simulink model "TeamA_PAsqualo"  (R2020a)
settings: Solver=VariableStepAuto  StartTime=0.0  StopTime=stop_time  FixedStep=0.05  RelTol=1e-3
InitFcn:
  | main_init
values from neighbouring files (symbols this model uses):
  a1 = rho * D^4 * alpha1    (= 0.000388302366464)    [main_init.m]
  a2 = -rho * D^3 * alpha2 * (1 - omega)    (= 0.0037030698432)    [main_init.m]
  ag = [Ax Ay Az]'    [init_modello.m]
  alpha1 = 0.0113    [main_init.m]
  alpha2 = -0.0091    [main_init.m]
  areaOfInterestCorner = [42.317744;10.915136; 0]    [init_controllo.m]    (also in missionA.m = [42.317744)
  bg = [Bx By Bz]'    [init_modello.m]
  cd_pitch = 0.7    [init_modello.m]
  cd_roll = 0.04    [init_modello.m]
  cd_x = 0.4    [init_modello.m]
  cd_y = 1    [init_modello.m]
  cd_yaw = 0.7    [init_modello.m]
  cd_z = 1    [init_modello.m]
  cg = [Cx Cy Cz]'    [init_modello.m]
  D = 0.076    [main_init.m]
  dead_zone_limit = 31.5    [main_init.m]
  dg = [Dx Dy Dz]'    [init_modello.m]
  eg = [Ex Ey Ez]'    [init_modello.m]
  fg = [Fx Fy Fz]'    [init_modello.m]
  g = 9.81    [init_modello.m]
  galleggiamento = 7.6786    [init_controllo.m]
  gg = [Gx Gy Gz]'    [init_modello.m]
  H0 = 0    [init_modello.m]
  init_position = [pointP(1),pointP(2),0.15,0,0,deg2rad(alpha)]'    [init_modello.m]
  init_velocity = [0 0 0 0 0 0]'    [init_modello.m]
  initial_state_cov = blkdiag(diag(cov_gps(1,1:2)), cov_depth*eye(n_state_filter-2))    [init_navigazione.m]
  Ixx = 0.93304097392    [init_modello.m]
  Ixy = 0    [init_modello.m]
  Ixz = 0    [init_modello.m]
  Iyy = 25.58745481378    (= 25.5874548138)    [init_modello.m]
  Iyz = 0    [init_modello.m]
  Izz = 25.58745481378    (= 25.5874548138)    [init_modello.m]
  K_i_heave_div = 20    [init_controllo.m]
  K_i_heave_pos = 1    [init_controllo.m]
  K_i_heave_surf = 20    [init_controllo.m]
  K_i_heave_trans = 5    [init_controllo.m]
  K_i_heave_turn = 5    [init_controllo.m]
  K_i_pitch_div = 0    [init_controllo.m]
  K_i_pitch_pos = 0    [init_controllo.m]
  K_i_pitch_surf = 0    [init_controllo.m]
  K_i_pitch_trans = 0    [init_controllo.m]
  K_i_pitch_turn = 0    [init_controllo.m]
  K_i_roll_div = 0    [init_controllo.m]
  K_i_roll_pos = 0    [init_controllo.m]
  K_i_roll_surf = 1    [init_controllo.m]
  K_i_roll_trans = 0    [init_controllo.m]
  K_i_roll_turn = 0    [init_controllo.m]
  K_i_surge_div = 3    [init_controllo.m]
  K_i_surge_pos = 5    [init_controllo.m]
  K_i_surge_surf = 3    [init_controllo.m]
  K_i_surge_trans = 2.5    [init_controllo.m]
  K_i_surge_turn = 10    [init_controllo.m]
  K_i_sway_div = 6    [init_controllo.m]
  K_i_sway_pos = 5    [init_controllo.m]
  K_i_sway_surf = 3    [init_controllo.m]
  K_i_sway_trans = 6    [init_controllo.m]
  K_i_sway_turn = 50    [init_controllo.m]
  K_i_yaw_div = 0    [init_controllo.m]
  K_i_yaw_pos = 1    [init_controllo.m]
  K_i_yaw_surf = 0    [init_controllo.m]
  K_i_yaw_trans = 20    [init_controllo.m]
  K_p_heave_div = 200    [init_controllo.m]
  K_p_heave_pos = 350    [init_controllo.m]
  K_p_heave_surf = 200    [init_controllo.m]
  K_p_heave_trans = 200    [init_controllo.m]
  K_p_heave_turn = 200    [init_controllo.m]
  K_p_phi_div = 0.15    [init_controllo.m]
  K_p_phi_pos = 0.1    [init_controllo.m]
  K_p_phi_surf = 0.15    [init_controllo.m]
  K_p_phi_trans = 0.1    [init_controllo.m]
  K_p_phi_turn = 0.1    [init_controllo.m]
  K_p_pitch_div = 50    [init_controllo.m]
  K_p_pitch_pos = 25    [init_controllo.m]
  K_p_pitch_surf = 50    [init_controllo.m]
  K_p_pitch_trans = 25    [init_controllo.m]
  K_p_pitch_turn = 25    [init_controllo.m]
  K_p_psi_div = 0.3    [init_controllo.m]
  K_p_psi_pos = 0.25    [init_controllo.m]
  K_p_psi_surf = 0.3    [init_controllo.m]
  K_p_psi_trans = 0.2    [init_controllo.m]
  K_p_roll_div = 10    [init_controllo.m]
  K_p_roll_pos = 4    [init_controllo.m]
  K_p_roll_surf = 10    [init_controllo.m]
  K_p_roll_trans = 4    [init_controllo.m]
  K_p_roll_turn = 4    [init_controllo.m]
  K_p_surge_div = 80    [init_controllo.m]
  K_p_surge_pos = 34.5    [init_controllo.m]
  K_p_surge_surf = 80    [init_controllo.m]
  K_p_surge_trans = 40    [init_controllo.m]
  K_p_surge_turn = 150    [init_controllo.m]
  K_p_sway_div = 100    [init_controllo.m]
  K_p_sway_pos = 90    [init_controllo.m]
  K_p_sway_surf = 80    [init_controllo.m]
  K_p_sway_trans = 90    [init_controllo.m]
  K_p_sway_turn = 200    [init_controllo.m]
  K_p_th_div = 0.3    [init_controllo.m]
  K_p_th_pos = 0.1    [init_controllo.m]
  K_p_th_surf = 0.3    [init_controllo.m]
  K_p_th_trans = 0.1    [init_controllo.m]
  K_p_th_turn = 0.1    [init_controllo.m]
  K_p_x_div = 0.12    [init_controllo.m]
  K_p_x_pos = 0.12    [init_controllo.m]
  K_p_x_surf = 0.12    [init_controllo.m]
  K_p_y_div = 0.6    [init_controllo.m]
  K_p_y_pos = 0.34    [init_controllo.m]
  K_p_y_surf = 0.1    [init_controllo.m]
  K_p_y_trans = 0.3    [init_controllo.m]
  K_p_y_turn = 0.3    [init_controllo.m]
  K_p_yaw_div = 70    [init_controllo.m]
  K_p_yaw_pos = 20    [init_controllo.m]
  K_p_yaw_surf = 70    [init_controllo.m]
  K_p_yaw_trans = 160    [init_controllo.m]
  K_p_z_div = 0.35    [init_controllo.m]
  K_p_z_pos = 0.2    [init_controllo.m]
  K_p_z_surf = 0.35    [init_controllo.m]
  K_p_z_trans = 0.7    [init_controllo.m]
  K_p_z_turn = 0.7    [init_controllo.m]
  Kadd = 0    [init_modello.m]
  m = 106    [init_modello.m]
  Madd = -((((1/5)*(b^2-a^2)^2))*(alpha_0-beta_0))/((((2*(b^2-a^2)^2))+(b^2-a^2)^2)*(alpha_0-beta_0)*m)    [init_modello.m]
  ... (+59 more)
undefined symbols (not defined in the file or in its folder): DiscIntNeverNeededParam, initial_state
libraries: simulink x2, vrlib x1
(part 3 of 5)

== system TeamA_PAsqualo/controller/surfacing controller/sway_controller/Sway PID controller ==
  enable : Inport
  references : Inport  Port=2
  "estimated measures " : Inport  Port=3
  Constant : Constant
  Constant1 : Constant  Value=0
  Discrete-Time Integrator : DiscreteIntegrator  ExternalReset=falling  SampleTime=0.1  ICPrevOutput=DiscIntNeverNeededParam  ICPrevScaledInput=DiscIntNeverNeededParam
  K_i_sway_surf : Gain  Gain=K_i_sway_surf
  K_p_sway_surf : Gain  Gain=K_p_sway_surf
  K_p_y_surf : Gain  Gain=K_p_y_surf
  Sum2 : Sum
  Switch : Switch  Threshold=1
  compute_position_errors : MATLAB Function  TreatAsAtomicUnit=on
  compute_velocity_error : MATLAB Function  TreatAsAtomicUnit=on
  Y : Outport
  wires:
  references/1 -> compute_position_errors/2(ref)
  compute_position_errors/1(err_pos) -> K_p_y_surf/1  "err_y"
  K_p_y_surf/1 -> compute_velocity_error/2(v_des)
  "estimated measures "/1 -> compute_velocity_error/3(est_meas), compute_position_errors/3(est_state)
  K_i_sway_surf/1 -> Discrete-Time Integrator/1
  K_p_sway_surf/1 -> Sum2/1
  Sum2/1 -> Y/1
  compute_velocity_error/1(err_vel) -> K_i_sway_surf/1, K_p_sway_surf/1  "err_vel"
  Discrete-Time Integrator/1 -> Sum2/2
  Switch/1 -> Discrete-Time Integrator/2
  enable/1 -> Switch/2, compute_velocity_error/1(enable), compute_position_errors/1(enable)
  Constant1/1 -> Switch/3
  Constant/1 -> Switch/1

== system TeamA_PAsqualo/controller/surfacing controller/yaw_controller/Yaw PID controller ==
  enable : Inport
  references : Inport  Port=2
  "estimated measures " : Inport  Port=3
  Constant : Constant
  Constant1 : Constant  Value=0
  Discrete-Time Integrator : DiscreteIntegrator  ExternalReset=falling  SampleTime=0.1  ICPrevOutput=DiscIntNeverNeededParam  ICPrevScaledInput=DiscIntNeverNeededParam
  K_i_yaw_surf : Gain  Gain=K_i_yaw_surf
  K_p_psi_surf : Gain  Gain=K_p_psi_surf
  K_p_yaw_surf : Gain  Gain=K_p_yaw_surf
  Sum2 : Sum
  Switch : Switch  Threshold=1
  compute_orientation_errors : MATLAB Function  TreatAsAtomicUnit=on
  compute_velocity_error : MATLAB Function  TreatAsAtomicUnit=on
  N : Outport
  wires:
  references/1 -> compute_orientation_errors/2(ref)
  "estimated measures "/1 -> compute_velocity_error/3(est_meas), compute_orientation_errors/3(est_state)
  compute_orientation_errors/1(err_orient) -> K_p_psi_surf/1  "err_orient"
  K_p_psi_surf/1 -> compute_velocity_error/2(v_des)
  Sum2/1 -> N/1
  Discrete-Time Integrator/1 -> Sum2/2
  K_i_yaw_surf/1 -> Discrete-Time Integrator/1
  K_p_yaw_surf/1 -> Sum2/1
  compute_velocity_error/1(err_vel) -> K_i_yaw_surf/1, K_p_yaw_surf/1  "err_vel"
  Switch/1 -> Discrete-Time Integrator/2
  enable/1 -> Switch/2, compute_velocity_error/1(enable), compute_orientation_errors/1(enable)
  Constant1/1 -> Switch/3
  Constant/1 -> Switch/1

== system TeamA_PAsqualo/controller/transect controller/heave_controller/Heave PID controller ==
  enable : Inport
  references : Inport  Port=2
  "estimated measures " : Inport  Port=3
  Constant : Constant  Value=galleggiamento
  Constant1 : Constant
  Constant2 : Constant  Value=0
  Discrete-Time Integrator : DiscreteIntegrator  ExternalReset=falling  InitialConditionSource=external  SampleTime=0.1  ICPrevOutput=DiscIntNeverNeededParam  ICPrevScaledInput=DiscIntNeverNeededParam
  K_i_heave_trans : Gain  Gain=K_i_heave_trans
  K_p_heave_trans : Gain  Gain=K_p_heave_trans
  K_p_z_trans : Gain  Gain=K_p_z_trans
  Sum2 : Sum
  Switch : Switch  Threshold=1
  compute_position_errors : MATLAB Function  TreatAsAtomicUnit=on
  compute_velocity_error : MATLAB Function  TreatAsAtomicUnit=on
  Z : Outport
  wires:
  "estimated measures "/1 -> compute_velocity_error/3(est_meas), compute_position_errors/3(est_state)
  K_p_z_trans/1 -> compute_velocity_error/2(v_des)
  compute_position_errors/1(err_pos) -> K_p_z_trans/1  "err_vect"
  references/1 -> compute_position_errors/2(ref)
  Sum2/1 -> Z/1
  Discrete-Time Integrator/1 -> Sum2/2
  K_p_heave_trans/1 -> Sum2/1
  K_i_heave_trans/1 -> Discrete-Time Integrator/1
  compute_velocity_error/1(err_vel) -> K_i_heave_trans/1, K_p_heave_trans/1  "err_vel"
  Constant/1 -> Discrete-Time Integrator/3
  Switch/1 -> Discrete-Time Integrator/2
  enable/1 -> Switch/2, compute_velocity_error/1(enable), compute_position_errors/1(enable)
  Constant2/1 -> Switch/3
  Constant1/1 -> Switch/1

== system TeamA_PAsqualo/controller/transect controller/pitch_controller/Pitch PID controller ==
  enable : Inport
  references : Inport  Port=2
  "estimated measures " : Inport  Port=3
  Constant : Constant
  Constant1 : Constant  Value=0
  Discrete-Time Integrator : DiscreteIntegrator  ExternalReset=falling  SampleTime=0.1  ICPrevOutput=DiscIntNeverNeededParam  ICPrevScaledInput=DiscIntNeverNeededParam
  K_i_pitch_trans : Gain  Gain=K_i_pitch_trans
  K_p_pitch_trans : Gain  Gain=K_p_pitch_trans
  K_p_th_trans : Gain  Gain=K_p_th_trans
  Sum2 : Sum
  Switch : Switch  Threshold=1
  compute_orientation_errors : MATLAB Function  TreatAsAtomicUnit=on
  compute_velocity_error : MATLAB Function  TreatAsAtomicUnit=on
  M : Outport
  wires:
  references/1 -> compute_orientation_errors/2(ref)
  K_p_th_trans/1 -> compute_velocity_error/2(v_des)
  "estimated measures "/1 -> compute_velocity_error/3(est_meas), compute_orientation_errors/3(est_state)
  compute_orientation_errors/1(err_orient) -> K_p_th_trans/1  "err_orient"
  Sum2/1 -> M/1
  Discrete-Time Integrator/1 -> Sum2/2
  K_p_pitch_trans/1 -> Sum2/1
  K_i_pitch_trans/1 -> Discrete-Time Integrator/1
  compute_velocity_error/1(err_vel) -> K_i_pitch_trans/1, K_p_pitch_trans/1  "err_vel"
  Switch/1 -> Discrete-Time Integrator/2
  enable/1 -> Switch/2, compute_velocity_error/1(enable), compute_orientation_errors/1(enable)
  Constant1/1 -> Switch/3
  Constant/1 -> Switch/1

== system TeamA_PAsqualo/controller/transect controller/roll_controller/Roll PID controller ==
  enable : Inport
  references : Inport  Port=2
  "estimated measures " : Inport  Port=3
  Constant : Constant
  Constant1 : Constant  Value=0
  Discrete-Time Integrator : DiscreteIntegrator  ExternalReset=falling  SampleTime=0.1  ICPrevOutput=DiscIntNeverNeededParam  ICPrevScaledInput=DiscIntNeverNeededParam
  K_i_roll_trans : Gain  Gain=K_i_roll_trans
  K_p_phi_trans : Gain  Gain=K_p_phi_trans
  K_p_roll_trans : Gain  Gain=K_p_roll_trans
  Sum2 : Sum
  Switch : Switch  Threshold=1
  compute_orientation_errors : MATLAB Function  TreatAsAtomicUnit=on
  compute_velocity_error : MATLAB Function  TreatAsAtomicUnit=on
  tau_roll : Outport
  wires:
  "estimated measures "/1 -> compute_velocity_error/3(est_meas), compute_orientation_errors/3(est_state)
  K_p_phi_trans/1 -> compute_velocity_error/2(v_des)
  compute_orientation_errors/1(err_orient) -> K_p_phi_trans/1  "err_orient"
  references/1 -> compute_orientation_errors/2(ref)
  Sum2/1 -> tau_roll/1
  Discrete-Time Integrator/1 -> Sum2/2
  K_p_roll_trans/1 -> Sum2/1
  K_i_roll_trans/1 -> Discrete-Time Integrator/1
  compute_velocity_error/1(err_vel) -> K_p_roll_trans/1, K_i_roll_trans/1  "err_vel"
  Switch/1 -> Discrete-Time Integrator/2
  Constant1/1 -> Switch/3
  Constant/1 -> Switch/1
  enable/1 -> Switch/2, compute_velocity_error/1(enable), compute_orientation_errors/1(enable)

== system TeamA_PAsqualo/controller/transect controller/surge_controller/Surge PID controller ==
  enable : Inport
  ref : Inport  Port=2
  est_meas : Inport  Port=3
  " compute_velocity_error" : MATLAB Function  TreatAsAtomicUnit=on
  Constant : Constant
  Constant1 : Constant  Value=0
  Discrete-Time Integrator : DiscreteIntegrator  ExternalReset=falling  SampleTime=0.1  ICPrevOutput=DiscIntNeverNeededParam  ICPrevScaledInput=DiscIntNeverNeededParam
  K_i_surge_trans : Gain  Gain=K_i_surge_trans
  K_p_surge_trans : Gain  Gain=K_p_surge_trans
  Scope : Scope
  Sum2 : Sum
  Switch : Switch  Threshold=1
  X : Outport
  wires:
  est_meas/1 -> " compute_velocity_error"/3(est_meas)
  ref/1 -> " compute_velocity_error"/2(ref)
  " compute_velocity_error"/1(err_vel) -> K_i_surge_trans/1, K_p_surge_trans/1  "err_vel"
  K_p_surge_trans/1 -> Sum2/1
  Sum2/1 -> Scope/1, X/1  "X"
  K_i_surge_trans/1 -> Discrete-Time Integrator/1
  Discrete-Time Integrator/1 -> Sum2/2
  Switch/1 -> Discrete-Time Integrator/2
  enable/1 -> Switch/2, " compute_velocity_error"/1(enable)
  Constant1/1 -> Switch/3
  Constant/1 -> Switch/1

== system TeamA_PAsqualo/controller/transect controller/sway_controller/Sway PID controller ==
  enable : Inport
  references : Inport  Port=2
  "estimated measures " : Inport  Port=3
  Constant : Constant
  Constant1 : Constant  Value=0
  Discrete-Time Integrator : DiscreteIntegrator  ExternalReset=falling  SampleTime=0.1  LimitOutput=on  ICPrevOutput=DiscIntNeverNeededParam  ICPrevScaledInput=DiscIntNeverNeededParam
  K_i_sway_trans : Gain  Gain=K_i_sway_trans
  K_p_sway_trans : Gain  Gain=K_p_sway_trans
  K_p_y_trans : Gain  Gain=K_p_y_trans
  Scope : Scope
  Sum2 : Sum
  Switch : Switch  Threshold=1
  compute_position_errors : MATLAB Function  TreatAsAtomicUnit=on
  compute_velocity_error : MATLAB Function  TreatAsAtomicUnit=on
  Y : Outport
  wires:
  references/1 -> compute_position_errors/2(ref)
  compute_position_errors/1(err_pos) -> K_p_y_trans/1  "err_vect"
  K_p_y_trans/1 -> compute_velocity_error/2(v_des)
  "estimated measures "/1 -> compute_velocity_error/3(est_meas), compute_position_errors/3(est_state)
  compute_velocity_error/1(err_vel) -> K_i_sway_trans/1, K_p_sway_trans/1  "err_vel"
  Discrete-Time Integrator/1 -> Scope/1, Sum2/2
  K_i_sway_trans/1 -> Discrete-Time Integrator/1
  Sum2/1 -> Y/1
  K_p_sway_trans/1 -> Sum2/1
  Switch/1 -> Discrete-Time Integrator/2
  enable/1 -> Switch/2, compute_velocity_error/1(enable), compute_position_errors/1(enable)
  Constant1/1 -> Switch/3
  Constant/1 -> Switch/1

== system TeamA_PAsqualo/controller/transect controller/yaw_controller/Yaw PID controller ==
  enable : Inport
  references : Inport  Port=2
  "estimated measures " : Inport  Port=3
  Constant : Constant
  Constant1 : Constant  Value=0
  Discrete-Time Integrator : DiscreteIntegrator  ExternalReset=falling  SampleTime=0.1  ICPrevOutput=DiscIntNeverNeededParam  ICPrevScaledInput=DiscIntNeverNeededParam
  K_i_yaw_trans : Gain  Gain=K_i_yaw_trans
  K_p_psi_trans : Gain  Gain=K_p_psi_trans
  K_p_yaw_trans : Gain  Gain=K_p_yaw_trans
  Sum2 : Sum
  Switch : Switch  Threshold=1
  compute_orientation_errors : MATLAB Function  TreatAsAtomicUnit=on
  compute_velocity_error : MATLAB Function  TreatAsAtomicUnit=on
  N : Outport
  wires:
  references/1 -> compute_orientation_errors/2(ref)
  "estimated measures "/1 -> compute_velocity_error/3(est_meas), compute_orientation_errors/3(est_state)
  compute_orientation_errors/1(err_orient) -> K_p_psi_trans/1  "err_orient"
  K_p_psi_trans/1 -> compute_velocity_error/2(v_des)
  Sum2/1 -> N/1
  Discrete-Time Integrator/1 -> Sum2/2
  K_p_yaw_trans/1 -> Sum2/1
  K_i_yaw_trans/1 -> Discrete-Time Integrator/1
  compute_velocity_error/1(err_vel) -> K_i_yaw_trans/1, K_p_yaw_trans/1  "err_vel"
  Switch/1 -> Discrete-Time Integrator/2
  enable/1 -> Switch/2, compute_velocity_error/1(enable), compute_orientation_errors/1(enable)
  Constant1/1 -> Switch/3
  Constant/1 -> Switch/1

== system TeamA_PAsqualo/controller/turning controller/heave_controller/Heave PID controller ==
  enable : Inport
  references : Inport  Port=2
  "estimated measures " : Inport  Port=3
  Constant : Constant  Value=galleggiamento
  Constant1 : Constant
  Constant2 : Constant  Value=0
  Discrete-Time Integrator : DiscreteIntegrator  ExternalReset=falling  InitialConditionSource=external  SampleTime=0.1  ICPrevOutput=DiscIntNeverNeededParam  ICPrevScaledInput=DiscIntNeverNeededParam
  K_i_heave_turn : Gain  Gain=K_i_heave_turn
  K_p_heave_turn : Gain  Gain=K_p_heave_turn
  K_p_z_turn : Gain  Gain=K_p_z_turn
  Sum2 : Sum
  Switch : Switch  Threshold=1
  compute_position_errors : MATLAB Function  TreatAsAtomicUnit=on
  compute_velocity_error : MATLAB Function  TreatAsAtomicUnit=on
  Z : Outport
  wires:
  "estimated measures "/1 -> compute_velocity_error/3(est_meas), compute_position_errors/3(est_state)
  K_p_z_turn/1 -> compute_velocity_error/2(v_des)
  compute_position_errors/1(err_pos) -> K_p_z_turn/1  "err_vect"
  references/1 -> compute_position_errors/2(ref)
  K_p_heave_turn/1 -> Sum2/1
  K_i_heave_turn/1 -> Discrete-Time Integrator/1
  Discrete-Time Integrator/1 -> Sum2/2
  Sum2/1 -> Z/1
  compute_velocity_error/1(err_vel) -> K_i_heave_turn/1, K_p_heave_turn/1  "err_vel"
  Constant/1 -> Discrete-Time Integrator/3
  Switch/1 -> Discrete-Time Integrator/2
  enable/1 -> Switch/2, compute_velocity_error/1(enable), compute_position_errors/1(enable)
  Constant2/1 -> Switch/3
  Constant1/1 -> Switch/1

== system TeamA_PAsqualo/controller/turning controller/pitch_controller/Pitch PID controller ==
  enable : Inport
  references : Inport  Port=2
  "estimated measures " : Inport  Port=3
  Constant : Constant
  Constant1 : Constant  Value=0
  Discrete-Time Integrator : DiscreteIntegrator  ExternalReset=falling  SampleTime=0.1  ICPrevOutput=DiscIntNeverNeededParam  ICPrevScaledInput=DiscIntNeverNeededParam
  K_i_pitch_turn : Gain  Gain=K_i_pitch_turn
  K_p_pitch_turn : Gain  Gain=K_p_pitch_turn
  K_p_th_turn : Gain  Gain=K_p_th_turn
  Sum2 : Sum
  Switch : Switch  Threshold=1
  compute_orientation_errors : MATLAB Function  TreatAsAtomicUnit=on
  compute_velocity_error : MATLAB Function  TreatAsAtomicUnit=on
  M : Outport
  wires:
  references/1 -> compute_orientation_errors/2(ref)
  K_p_th_turn/1 -> compute_velocity_error/2(v_des)
  "estimated measures "/1 -> compute_velocity_error/3(est_meas), compute_orientation_errors/3(est_state)
  compute_orientation_errors/1(err_orient) -> K_p_th_turn/1  "err_orient"
  Sum2/1 -> M/1
  compute_velocity_error/1(err_vel) -> K_i_pitch_turn/1, K_p_pitch_turn/1  "err_vel"
  Discrete-Time Integrator/1 -> Sum2/2
  K_p_pitch_turn/1 -> Sum2/1
  K_i_pitch_turn/1 -> Discrete-Time Integrator/1
  Switch/1 -> Discrete-Time Integrator/2
  enable/1 -> Switch/2, compute_velocity_error/1(enable), compute_orientation_errors/1(enable)
  Constant1/1 -> Switch/3
  Constant/1 -> Switch/1

== system TeamA_PAsqualo/controller/turning controller/roll_controller/Roll PID controller ==
  enable : Inport
  references : Inport  Port=2
  "estimated measures " : Inport  Port=3
  Constant : Constant
  Constant1 : Constant  Value=0
  Discrete-Time Integrator : DiscreteIntegrator  ExternalReset=falling  SampleTime=0.1  ICPrevOutput=DiscIntNeverNeededParam  ICPrevScaledInput=DiscIntNeverNeededParam
  K_i_roll_turn : Gain  Gain=K_i_roll_turn
  K_p_phi_turn : Gain  Gain=K_p_phi_turn
  K_p_roll_turn : Gain  Gain=K_p_roll_turn
  Sum2 : Sum
  Switch : Switch  Threshold=1
  compute_orientation_errors : MATLAB Function  TreatAsAtomicUnit=on
  compute_velocity_error : MATLAB Function  TreatAsAtomicUnit=on
  K : Outport
  wires:
  "estimated measures "/1 -> compute_velocity_error/3(est_meas), compute_orientation_errors/3(est_state)
  K_p_phi_turn/1 -> compute_velocity_error/2(v_des)
  compute_orientation_errors/1(err_orient) -> K_p_phi_turn/1  "err_orient"
  references/1 -> compute_orientation_errors/2(ref)
  Sum2/1 -> K/1
  compute_velocity_error/1(err_vel) -> K_i_roll_turn/1, K_p_roll_turn/1  "err_vel"
  Discrete-Time Integrator/1 -> Sum2/2
  K_p_roll_turn/1 -> Sum2/1
  K_i_roll_turn/1 -> Discrete-Time Integrator/1
  Switch/1 -> Discrete-Time Integrator/2
  enable/1 -> Switch/2, compute_velocity_error/1(enable), compute_orientation_errors/1(enable)
  Constant1/1 -> Switch/3
  Constant/1 -> Switch/1

== system TeamA_PAsqualo/controller/turning controller/surge_controller/Surge PID controller ==
  enable : Inport
  ref : Inport  Port=2
  est_meas : Inport  Port=3
  " compute_velocity_error" : MATLAB Function  TreatAsAtomicUnit=on
  Constant : Constant
  Constant1 : Constant  Value=0
  Constant2 : Constant  Value=turning_surge
  Discrete-Time Integrator : DiscreteIntegrator  ExternalReset=falling  InitialConditionSource=external  SampleTime=0.1  ICPrevOutput=DiscIntNeverNeededParam  ICPrevScaledInput=DiscIntNeverNeededParam
  K_i_surge_turn : Gain  Gain=K_i_surge_turn
  K_p_surge_turn : Gain  Gain=K_p_surge_turn
  Scope : Scope
  Sum2 : Sum
  Switch : Switch  Threshold=1
  X : Outport
  wires:
  est_meas/1 -> " compute_velocity_error"/3(est_meas)
  ref/1 -> " compute_velocity_error"/2(ref)
  Sum2/1 -> Scope/1, X/1
  Discrete-Time Integrator/1 -> Sum2/2
  K_p_surge_turn/1 -> Sum2/1
  K_i_surge_turn/1 -> Discrete-Time Integrator/1
  " compute_velocity_error"/1(err_vel) -> K_i_surge_turn/1, K_p_surge_turn/1  "err_vel"
  Switch/1 -> Discrete-Time Integrator/2
  enable/1 -> Switch/2, " compute_velocity_error"/1(enable)
  Constant1/1 -> Switch/3
  Constant/1 -> Switch/1
  Constant2/1 -> Discrete-Time Integrator/3

== system TeamA_PAsqualo/controller/turning controller/sway_controller/Sway PID controller ==
  enable : Inport
  references : Inport  Port=2
  "estimated measures " : Inport  Port=3
  Constant : Constant
  Constant1 : Constant  Value=0
  Discrete-Time Integrator : DiscreteIntegrator  ExternalReset=falling  SampleTime=0.1  ICPrevOutput=DiscIntNeverNeededParam  ICPrevScaledInput=DiscIntNeverNeededParam
  K_i_sway_turn : Gain  Gain=K_i_sway_turn
  K_p_sway_turn : Gain  Gain=K_p_sway_turn
  K_p_y_turn : Gain  Gain=K_p_y_turn
  Scope : Scope
  Sum2 : Sum
  Switch : Switch  Threshold=1
  compute_position_errors : MATLAB Function  TreatAsAtomicUnit=on
  compute_velocity_error : MATLAB Function  TreatAsAtomicUnit=on
  Y : Outport
  wires:
  references/1 -> compute_position_errors/2(ref)
  compute_position_errors/1(err_pos) -> K_p_y_turn/1  "err_vect"
  K_p_y_turn/1 -> compute_velocity_error/2(v_des)
  "estimated measures "/1 -> compute_velocity_error/3(est_meas), compute_position_errors/3(est_state)
  K_p_sway_turn/1 -> Sum2/1
  K_i_sway_turn/1 -> Discrete-Time Integrator/1
  Discrete-Time Integrator/1 -> Scope/1, Sum2/2
  compute_velocity_error/1(err_vel) -> K_i_sway_turn/1, K_p_sway_turn/1  "err_vel"
  Sum2/1 -> Y/1
  Switch/1 -> Discrete-Time Integrator/2
  enable/1 -> Switch/2, compute_velocity_error/1(enable), compute_position_errors/1(enable)
  Constant1/1 -> Switch/3
  Constant/1 -> Switch/1

== system TeamA_PAsqualo/controller/turning controller/yaw_controller/Yaw PID controller ==
  enable : Inport
  ref : Inport  Port=2
  est_meas : Inport  Port=3
  Constant2 : Constant
  Constant3 : Constant  Value=0
  Discrete-Time Integrator1 : DiscreteIntegrator  ExternalReset=falling  SampleTime=0.1  ICPrevOutput=DiscIntNeverNeededParam  ICPrevScaledInput=DiscIntNeverNeededParam
  K_i_yaw_trans : Gain  Gain=K_i_yaw_trans
  K_p_psi_trans : Gain  Gain=K_p_psi_trans
  K_p_yaw_trans : Gain  Gain=K_p_yaw_trans
  Sum1 : Sum
  Switch1 : Switch  Threshold=1
  compute_orientation_errors : MATLAB Function  TreatAsAtomicUnit=on
  compute_velocity_error : MATLAB Function  TreatAsAtomicUnit=on
  N : Outport
  wires:
  Constant3/1 -> Switch1/3
  Constant2/1 -> Switch1/1
  K_p_psi_trans/1 -> compute_velocity_error/2(v_des)
  Switch1/1 -> Discrete-Time Integrator1/2
  compute_velocity_error/1(err_vel) -> K_i_yaw_trans/1, K_p_yaw_trans/1  "err_vel"
  enable/1 -> Switch1/2, compute_velocity_error/1(enable), compute_orientation_errors/1(enable)
  K_i_yaw_trans/1 -> Discrete-Time Integrator1/1
  compute_orientation_errors/1(err_orient) -> K_p_psi_trans/1  "err_orient"
  est_meas/1 -> compute_orientation_errors/3(est_state), compute_velocity_error/3(est_meas)
  K_p_yaw_trans/1 -> Sum1/1
  ref/1 -> compute_orientation_errors/2(ref)
  Discrete-Time Integrator1/1 -> Sum1/2
  Sum1/1 -> N/1

== matlab function TeamA_PAsqualo/Vehicle Model/J1 computation ==
  data: eta input; J1 output
function J1 = fcn(eta)
phi = eta(4);
theta = eta(5);
psi = eta(6);
Rx = [1 0 0;0 cos(phi) sin(phi);0 -sin(phi) cos(phi)];
Ry = [cos(theta) 0 -sin(theta);0 1 0;sin(theta) 0 cos(theta)];
Rz = [cos(psi) sin(psi) 0;-sin(psi) cos(psi) 0; 0 0 1];
J1 = Rz'*Ry'*Rx';
end

== matlab function TeamA_PAsqualo/Vehicle Model/ni_dot computation ==
  data: M_times_nir_dot input double size=[6 1]; nir_dot output double size=[6 1]; M_inv parameter
function nir_dot = fcn(M_times_nir_dot, M_inv)
nir_dot = M_inv * M_times_nir_dot;
end

== matlab function TeamA_PAsqualo/Vehicle Model/ni_to_eta_dot ==
  data: J input; ni_abs input; eta_dot output
function eta_dot = fcn(J,ni_abs)
eta_dot = J*ni_abs;
end

== matlab function TeamA_PAsqualo/Sensors and Environment Models /Global Positioning System/WGS84toNed  ==
  data: posizione input; posizione_NED output
function posizione_NED = wgs84toNed(posizione)

coder.extrinsic('evalin', 'wgs84Ellipsoid', 'geodetic2ned');
NED_origin = [0;0;0];
posizione_NED  = [0;0;0];
NED_origin = evalin('base', 'NED_origin');
[a, b, c] = geodetic2ned(posizione(1), posizione(2), posizione(3), NED_origin(1), NED_origin(2), NED_origin(3), wgs84Ellipsoid);
posizione_NED = [a; b; posizione(3)];

end

== matlab function TeamA_PAsqualo/Sensors and Environment Models /Profondimetro/WGS84toNed  ==
  data: posizione input; posizione_NED output
function posizione_NED = wgs84toNed(posizione)

coder.extrinsic('evalin', 'wgs84Ellipsoid', 'geodetic2ned');
NED_origin = [0;0;0];
posizione_NED  = [0;0;0];
NED_origin = evalin('base', 'NED_origin');
[a, b, c] = geodetic2ned(posizione(1), posizione(2), posizione(3), NED_origin(1), NED_origin(2), NED_origin(3), wgs84Ellipsoid);
posizione_NED = [a; b; posizione(3)];

end

== matlab function TeamA_PAsqualo/Sensors and Environment Models /Sonar_down/MATLAB Function ==
  data: posizione input; p_sonar_ned output; orientazione input; s_versor_ned output; tilt input; p_sonar_body input
function [p_sonar_ned, s_versor_ned] = rot_body_ned(posizione,orientazione,tilt,p_sonar_body)
   
 roll = orientazione(1);
 pitch = orientazione(2);
 yaw = orientazione(3);
 xNorth = posizione(1);
 yEast = posizione(2);
 zDown = posizione(3);
 Rx = [1 0 0; 0 cos(roll) -sin(roll); 0 sin(roll) cos(roll)];
 Ry = [cos(pitch) 0 sin(pitch); 0 1 0; -sin(pitch) 0 cos(pitch)];
 Rz = [cos(yaw) -sin(yaw) 0; sin(yaw) cos(yaw) 0; 0 0 1];
 J1 = Rz*Ry*Rx; %matrice di rotazione da body a ned frame 

 s_versor_body = [sin(tilt); 0 ; cos(tilt)];	% direzione sonar in terna body
 s_versor_ned = J1*s_versor_body;
 
 cs2sensor_ned = J1*p_sonar_body; % distanza cds-sensore in Ned
 %Posizione sensore in Ned frame:
 p_sonar_ned = [xNorth; yEast; zDown] + cs2sensor_ned;
end

== matlab function TeamA_PAsqualo/Sensors and Environment Models /Sonar_down/MATLAB Function1 ==
  data: p_sonar_ned input; sol_t output; s_versor_ned input
function sol_t = sonar_down(p_sonar_ned, s_versor_ned)

coder.extrinsic('seabed_function');
sol_t = 0;
sol_t = seabed_function(p_sonar_ned, s_versor_ned);

end

== matlab function TeamA_PAsqualo/Sensors and Environment Models /Sonar_down/WGS84toNed 1 ==
  data: posizione input; posizione_NED output
function posizione_NED = wgs84toNed(posizione)

coder.extrinsic('evalin', 'wgs84Ellipsoid', 'geodetic2ned');
NED_origin = [0;0;0];
posizione_NED  = [0;0;0];
NED_origin = evalin('base', 'NED_origin');
[a, b, c] = geodetic2ned(posizione(1), posizione(2), posizione(3), NED_origin(1), NED_origin(2), NED_origin(3), wgs84Ellipsoid);
posizione_NED = [a; b; posizione(3)];

end

== matlab function TeamA_PAsqualo/Sensors and Environment Models /Sonar_front/MATLAB Function ==
  data: posizione input; p_sonar_ned output; orientazione input; s_versor_ned output; tilt input; p_sonar_body input
function [p_sonar_ned, s_versor_ned] = rot_body_ned(posizione,orientazione,tilt,p_sonar_body)
   
 roll = orientazione(1);
 pitch = orientazione(2);
 yaw = orientazione(3);
 xNorth = posizione(1);
 yEast = posizione(2);
 zDown = posizione(3);
 Rx = [1 0 0; 0 cos(roll) -sin(roll); 0 sin(roll) cos(roll)];
 Ry = [cos(pitch) 0 sin(pitch); 0 1 0; -sin(pitch) 0 cos(pitch)];
 Rz = [cos(yaw) -sin(yaw) 0; sin(yaw) cos(yaw) 0; 0 0 1];
 J1 = Rz*Ry*Rx; %matrice di rotazione da body a ned frame 

 s_versor_body = [sin(tilt); 0 ; cos(tilt)];	% direzione sonar in terna body
 s_versor_ned = J1*s_versor_body;
 
 cs2sensor_ned = J1*p_sonar_body; % distanza cds-sensore in Ned
 %Posizione sensore in Ned frame:
 p_sonar_ned = [xNorth; yEast; zDown] + cs2sensor_ned;
end

== matlab function TeamA_PAsqualo/Sensors and Environment Models /Sonar_front/MATLAB Function1 ==
  data: p_sonar_ned input; sol_t output; s_versor_ned input
function sol_t = sonar_down(p_sonar_ned, s_versor_ned)

coder.extrinsic('seabed_function');
sol_t = 0;
sol_t = seabed_function(p_sonar_ned, s_versor_ned);

end

== matlab function TeamA_PAsqualo/Sensors and Environment Models /Sonar_front/WGS84toNed 1 ==
  data: posizione input; posizione_NED output
function posizione_NED = wgs84toNed(posizione)

coder.extrinsic('evalin', 'wgs84Ellipsoid', 'geodetic2ned');
NED_origin = [0;0;0];
posizione_NED  = [0;0;0];
NED_origin = evalin('base', 'NED_origin');
[a, b, c] = geodetic2ned(posizione(1), posizione(2), posizione(3), NED_origin(1), NED_origin(2), NED_origin(3), wgs84Ellipsoid);
posizione_NED = [a; b; posizione(3)];

end

== matlab function TeamA_PAsqualo/Sensors and Environment Models /Ultra Short Base Line System/MATLAB Function1 ==
  data: x_t_usbl input; bearing output; y_t_usbl input; z_t_usbl input; elevation output; range output
function [bearing,elevation,range] = usbl(x_t_usbl, y_t_usbl, z_t_usbl)
%coordinate sferiche in uscita dal sensore
range = sqrt((x_t_usbl)^2+(y_t_usbl)^2+(z_t_usbl^2)); 
elevation = asin(z_t_usbl/range);
bearing = atan2(y_t_usbl,x_t_usbl); 

 end

== matlab function TeamA_PAsqualo/Sensors and Environment Models /Ultra Short Base Line System/MATLAB Function2 ==
  data: posizione input; x_t_usbl output; orientazione input; p_usbl input; p_transponder input; y_t_usbl output; z_t_usbl output
function [x_t_usbl,y_t_usbl,z_t_usbl]= rot_ned_usbl(posizione,orientazione, p_usbl, p_transponder)
 
roll = orientazione(1);
pitch = orientazione(2);
yaw = orientazione(3);
xNorth = posizione(1);
yEast = posizione(2);
zDown = posizione(3);
Rx = [1 0 0; 0 cos(roll) -sin(roll); 0 sin(roll) cos(roll)];
Ry = [cos(pitch) 0 sin(pitch); 0 1 0; -sin(pitch) 0 cos(pitch)];
Rz = [cos(yaw) -sin(yaw) 0; sin(yaw) cos(yaw) 0; 0 0 1];
J1 = Rz*Ry*Rx; %matrice di rotazione da body a ned frame 
p_usbl_ned = J1*p_usbl; % offset sensore -centro di simmetria riportato in terna ned 
p_sensore = p_usbl_ned + [xNorth;yEast;zDown]; %posizione sensore in
% terna ned 
b2transp_ned = p_transponder - p_sensore; %distanza trasponder-usbl in terna ned 
x_t_usbl = b2transp_ned(1);
y_t_usbl = b2transp_ned(2);
z_t_usbl = b2transp_ned(3);

end

== matlab function TeamA_PAsqualo/Sensors and Environment Models /Ultra Short Base Line System/WGS84toNed 1 ==
  data: posizione input; posizione_NED output
function posizione_NED = wgs84toNed(posizione)

coder.extrinsic('evalin', 'wgs84Ellipsoid', 'geodetic2ned');
NED_origin = [0;0;0];
posizione_NED  = [0;0;0];
NED_origin = evalin('base', 'NED_origin');
[a, b, c] = geodetic2ned(posizione(1), posizione(2), posizione(3), NED_origin(1), NED_origin(2), NED_origin(3), wgs84Ellipsoid);
posizione_NED = [a; b; posizione(3)];

end

== matlab function TeamA_PAsqualo/Navigazione/Correzione/MATLAB Function ==
  settings: updateMethod=DISCRETE
  data: col output size=[1 5]; u input; row output size=[1 5]; run output
function [col ,row, run] = select(u)

    run = 0;
    row = [];
    col = [];
    
    if u(1) == 1 % gps
        row = [row 1 2];
        col = [col 1 2];
        run = 1;
    end
    if u(2) == 1 % usbl
        row = [row 3 4];
        col = [col 3 4];
        run = 1;
    end
    if u(3) == 1 % depth
        row = [row 5];
        col = [col 5];
        run = 1;
    end

   
end

== matlab function TeamA_PAsqualo/Navigazione/Correzione/MATLAB Function1 ==
  data: y_true input size=[n_meas_filter 1]; e output size=[n_meas_filter 1]; y_virt input size=[n_meas_filter 1]; select input
function e = innov_calc(y_true, y_virt, select)
% innov calc

e = y_true - y_virt;

% se e` pronta la misura dell'usbl,  calcolo
if select(2) == 1
	index = 2*select(1)+1;
	e(index,1) = atan2(sin(e(index,1)), cos(e(index,1)));
end


end

== matlab function TeamA_PAsqualo/Navigazione/Correzione/kalman correction ==
  data: x_old input; x_new output size=[3 1]; P_old input; e input size=[n_meas_filter 1]; P_new output; S input size=[n_meas_filter n_meas_filter]; C input size=[n_state_filter n_meas_filter]
function [x_new, P_new]= kalman_correction(x_old, P_old, e, S, C)

	K = C*(S^-1); 
    P_delta = - K*S*K';
	
    x_new = x_old + K*e;
    P = P_old + P_delta;    
	
	P_new = (P+P')/2;
end

== matlab function TeamA_PAsqualo/Navigazione/Predizione/predizione_propagate ==
  data: mean input size=[n_state_aug_filter 1]; mean_new output size=[n_state_filter, 1]; cov input size=[n_state_aug_filter n_state_aug_filter]; cov_new output size=[n_state_filter n_state_filter]; n_state_aug_filter parameter; ts_filter parameter; n_state_filter parameter
function [mean_new, cov_new] = propagate(mean, cov, n_state_aug_filter, ts_filter, n_state_filter)
 % PROPAGATE genera un numero n di sigma points, li propaga attraverso
 % state_update e da` come output la media e la covarianza dei nuovi sigma
 % points. 
 %
 % Input		
 % mean			vettore media dello stato nx1
 % cov			matrice covarianza dello stato nxn
 %
 % Output
 % mean_new		vettore media dello stato nx1
 % cov_new		matrice covarianza dello stato nxn

[sp, wm, wc] = sigmapoint_gen(mean, cov, n_state_aug_filter);

[mean_new, P] = sigmapoint_propagate(sp, wm, wc, ...
					n_state_aug_filter, ts_filter, n_state_filter);

% check simmetria
cov_new = (P + P')/2;

end

%--------------------------------------------------------------------------
%--------------------------------------------------------------------------
function state_new = state_update(state_aug, ts_filter)


pos = state_aug(1:3, 1);
ahrs = state_aug(4:6, 1); % roll pitch yaw
dvl = state_aug(7:9, 1);

% yaw, pitch, roll
Rbn = rotz(ahrs(3))' * roty(ahrs(2))' * rotx(ahrs(1))';

state_new = pos + ts_filter * Rbn * dvl;

end

function Rx = rotx(ang)

Rx = [	1 0 0; ...
		0 cos(ang) sin(ang); ...
		0 -sin(ang) cos(ang)];

end
function Ry = roty(ang)

Ry = [	cos(ang) 0 -sin(ang); ...
		0 1 0; ...
		sin(ang) 0 cos(ang)];

end
function Rz = rotz(ang)

Rz = [	cos(ang) sin(ang) 0; ...
		-sin(ang) cos(ang) 0; ...
		0	0 1];

end
		
%--------------------------------------------------------------------------
%--------------------------------------------------------------------------
function [sp, wm, wc] = sigmapoint_gen(mean, cov, n_state_filter)
% questa funzione genera i sigma point e i loro pesi
	

	n		= n_state_filter;	% Dimensione dello spazio in cui vengono generati
	nsp		= 2*n+1;			% numero di sigma points. in generale pari a (2n+1)
	P       = cov;				% matrice di covarianza
%	mean    = mean;				%
	
	% par da rivedere
	alpha	= 1;
	beta	= 2;
	k		= 0;
    
	%   
	lambda = alpha^2 * (n + k) -n;
	
	% generazione pesi per media
	wm = 1/(2*(n + lambda)) * ones(nsp, 1);
    wm(1) = lambda/(n + lambda);
	
	% generazione pesi per cov
	wc = 1/(2*(n + lambda)) * ones(nsp, 1);
	wc(1) = lambda/(n + lambda) + (1 - alpha^2 + beta);
	
	% generazione sigma points sp
	dist = zeros(n_state_filter,n_state_filter);
	sp = zeros(n_state_filter, nsp);
	
	[U, SIGMA, ~] = svd((n+lambda)* P);
	dist = U * sqrt(SIGMA);

	for i=1:nsp
		if i == 1
			sp(:,i) = mean;
		elseif i<=1+n
			sp(:,i) = mean+dist(:,i-1);
		elseif i>1+n && i<=nsp
			sp(:,i) = mean-dist(:,i-1-n);
		end
	end

end

%--------------------------------------------------------------------------
%--------------------------------------------------------------------------
function [mean_new, cov_new] = sigmapoint_propagate(sp, wm, wc, n_state_aug_filter, ts_filter, n_state_filter)
% questa funzione propaga i sigma point usando state_update
	
	
	nsp = n_state_aug_filter*2 + 1;
	sp_new = zeros(n_state_filter, nsp);
	for j = 1:nsp
		 sp_new(:,j) = state_update(sp(:,j), ts_filter);
	end

	% media
	mean_new = zeros(n_state_filter, 1);
	for j = 1:nsp
		mean_new = mean_new + wm(j)*sp_new(:,j);
	end

	% cov
	cov_new = zeros(n_state_filter, n_state_filter);  
	for j = 1:nsp
		 cov_new = cov_new + wc(j)*(sp_new(:,j) - mean_new)*(sp_new(:,j) - mean_new)';
	end

	
end

== matlab function TeamA_PAsqualo/Navigazione/Predizione/smart_mux ==
  data: x_mean input size=[n_state_filter 1]; mean output size=[9 1]; x_cov input size=[n_state_filter n_state_filter]; u_mean input size=[n_input_filter 1]; u_cov input size=[n_input_filter n_input_filter]; cov output size=[n_state_aug_filter, n_state_aug_filter]; n_state_filter parameter; n_input_filter parameter
function [mean, cov] = smart_mux(x_mean, x_cov, u_mean, u_cov, n_state_filter, n_input_filter)

% init
mean = zeros(n_state_filter+n_input_filter, 1);
mean = [x_mean; u_mean];
    
cov = zeros(n_state_filter + n_input_filter);
cov = blkdiag(x_cov, u_cov);

end

== matlab function TeamA_PAsqualo/Navigazione/Predizione Misure/propagazione misura NED1 ==
  data: x input; P input; y_virt output size=[5 1]; S_virt output; C output; n_state_filter parameter; n_meas_filter parameter; pos_transp parameter; p_usbl parameter; or input
function [y_virt, S_virt, C] = propagazione_misure(x, P, n_state_filter, n_meas_filter, pos_transp, p_usbl, or)
 % PROPAGATE_MISURE genera i sigma points, li propaga attraverso state2meas
 % e da` come output la media, la covarianza dei nuovi sigma points e la 
 % crosscovarianza stato-meas.
 %
 % Input		
 % mean			vettore media dello stato nx1
 % cov			matrice covarianza dello stato nxn
 %
 % Output
 % mean_new		vettore media dello misure mx1
 % cov_new		matrice covarianza dello delle misure mxm
 % C			matrice crosscovarianza nxm


[sp, wm, wc] = sigmapoint_gen(x, P, n_state_filter);

[~, y_virt, esse, C] = sigmapoint_propagate(sp, x, wm, wc, n_state_filter, ...
									n_meas_filter, pos_transp, p_usbl, or);

% check simmetria								
S_virt = (esse + esse')/2;


end

%--------------------------------------------------------------------------
%--------------------------------------------------------------------------
function meas = state2meas(state, n_meas_filter, pos_transp,  p_usbl, or)

meas = zeros(n_meas_filter,1);

Rbn = rotz(or(3))' * roty(or(2))' * rotx(or(1))';

% ned2usbl
pos_sensore_onboard = state(1:3,1) + Rbn*p_usbl;

vettore_auv_trasp =  +(pos_transp - pos_sensore_onboard) ;
range	= norm(vettore_auv_trasp,2);
bear	= atan2(vettore_auv_trasp(2),vettore_auv_trasp(1));

% depth
meas_depth = state(3);


meas = [state(1); state(2); bear; range; meas_depth];

end


function Rx = rotx(ang)

Rx = [	1 0 0; ...
		0 cos(ang) sin(ang); ...
		0 -sin(ang) cos(ang)];

end
function Ry = roty(ang)

Ry = [	cos(ang) 0 -sin(ang); ...
		0 1 0; ...
		sin(ang) 0 cos(ang)];

end
function Rz = rotz(ang)

Rz = [	cos(ang) sin(ang) 0; ...
		-sin(ang) cos(ang) 0; ...
		0	0 1];

end

%--------------------------------------------------------------------------
%--------------------------------------------------------------------------
function [sp, wm, wc] = sigmapoint_gen(mean, cov, n_state_filter)
% questa funzione genera i sigma point e i loro pesi


	n		= n_state_filter;	% Dimensione dello spazio in cui vengono generati
	nsp		= 2*n+1;			% numero di sigma points. in generale pari a (2n+1)
	P       = cov;				% matrice di covarianza
%	mean    = mean;				%
	
	% par da rivedere
	alpha	= 1;
	beta	= 2;
	k		= 0;
    
	%   
	lambda = alpha^2 * (n + k) -n;
	
	% generazione pesi per media
	wm = 1/(2*(n + lambda)) * ones(nsp, 1);
    wm(1) = lambda/(n + lambda);
	
	% generazione pesi per cov
	wc = 1/(2*(n + lambda)) * ones(nsp, 1);
	wc(1) = lambda/(n + lambda) + (1 - alpha^2 + beta);
	
	% generazione sigma points sp
	[U, SIGMA, ~] = svd((n+lambda)* P);
	dist = U * sqrt(SIGMA);
	
	sp = zeros(n_state_filter, nsp);
	for i=1:nsp
		if i == 1
			sp(:,i) = mean;
		elseif i<=1+n
			sp(:,i) = mean+dist(:,i-1);
		elseif i>1+n && i<=nsp
			sp(:,i) = mean-dist(:,i-1-n);
		end
	end
	%sp = [mean mean+dist(:,1) mean+dist(:,2) mean-dist(:,1) mean-dist(:,2)];
	%sp = [mean mean+dist mean-dist];

end

%--------------------------------------------------------------------------
%--------------------------------------------------------------------------
function [sp_new, mean_new, cov_new, C] = sigmapoint_propagate(sp, mean, wm, wc, n_state_filter, n_meas_filter, pos_transp, p_usbl, or)
% questa funzione propaga i sigma point usando state_update

	nsp = n_state_filter*2 + 1;
	
	sp_new = zeros(n_meas_filter, nsp);
	
	for j = 1:nsp
		%	state2meas(state, n_state_filter, n_meas_filter, ned_origin, spheroid)
		sp_new(:,j) = state2meas(sp(:,j), n_meas_filter,...
						pos_transp, p_usbl, or);
	end

	% media
	mean_new = mean_func(n_meas_filter, sp_new, wm, nsp);

	% cov
	[cov_new, C] = cov_func(sp, mean, sp_new, mean_new, wc, nsp, n_meas_filter, n_state_filter);
	
end

%--------------------------------------------------------------------------
%--------------------------------------------------------------------------
function mean_new = mean_func(n_meas_filter, sp_new, wm, nsp)
% ymeas = 	lat
% 			lon
% 			bear
% 			range
% 			depth

mean_new = zeros(n_meas_filter, 1);

for j = 1:nsp
	mean_new = mean_new + wm(j)*sp_new(:,j);
end

%calcolo media bearing :)
mean_c = 0;
mean_s = 0;
for j = 1:nsp
	c = cos(sp_new(3,j));
	s = sin(sp_new(3,j));
	
	mean_c = mean_c + wm(j)*c;
	mean_s = mean_s + wm(j)*s;
end
mean_new(3) = atan2(mean_s, mean_c);

end

%--------------------------------------------------------------------------
%--------------------------------------------------------------------------
function [cov_new, C] = cov_func(sp, mean, sp_new, mean_new, wc, nsp, n_meas_filter, n_state_filter)
% ymeas = 	lat
% 			lon
% 			bear
% 			range
% 			depth

% init
cov_new = zeros(n_meas_filter, n_meas_filter);  

C = zeros(n_state_filter, n_meas_filter);


% covarianza uscite non angolari
b = zeros(n_meas_filter, 1);
for j = 1:nsp
    b = sp_new(:,j) - mean_new(:,1);
    cov_new = cov_new + wc(j) * (b*b');
end

%covarianza bearing
cc = 0;
cs = 0;
for j = 1:nsp
	c = cos(sp_new(3,j) - mean_new(3));
	s = sin(sp_new(3,j) - mean_new(3));
	
	cc = cc + wc(j)*(c*c');
	cs = cs + wc(j)*(s*s');
end
cov_new(3,3) = atan2(cs,cc);


%----------------------------------------------------
% Calcolo Crosscovarianza
% 
% [	x1y1 x1y2 x1y3 x1y4 x1y5;
% 	x2y1 x2y2 x2y3 x2y4 x2y5;
% 	x3y1 x3y2 x3y3 x3y4 x3y5 
%	x4y1 x4y2 x4y3 x4y4 x4y5]

C = zeros(n_state_filter, n_meas_filter);
for j = 1:nsp
	
	C = C + wc(j)*((sp(:,j)-mean)*(sp_new(:,j) ...
								- mean_new(:,1))');
end

%covarianza bearing 
Cb = zeros(n_state_filter,1);
for j = 1:nsp
	ang = sp_new(3,j)- mean_new(3,1);
	a = atan2(sin(ang),cos(ang));
	Cb = Cb + wc(j)*((sp(:,j)-mean)*a);
end
C(:,3) = Cb;
end

== matlab function TeamA_PAsqualo/Navigazione/Selettore Misure/Selettore misure/MATLAB Function ==
  settings: updateMethod=DISCRETE
  data: col output size=[1 5]; u input; row output size=[1 5]; run output
function [col ,row, run] = select(u)

    run = 0;
    row = [];
    col = [];
    
    if u(1) == 1 % gps
        row = [row 1 2];
        col = [col 1 2];
        run = 1;
    end
    if u(2) == 1 % usbl
        row = [row 3 4];
        col = [col 3 4];
        run = 1;
    end
    if u(3) == 1 % depth
        row = [row 5];
        col = [col 5];
        run = 1;
    end

   
end

== matlab function TeamA_PAsqualo/Navigazione/Selettore Misure/Selettore misure/pulse/MATLAB Function ==
  data: gps_now input size=[2,1]; u input; y output; ned_origin parameter
function y  = tolo_pulse(gps_now,u, ned_origin)
% questa funzione fornisce 1 se il valore in ingresso e` cambiato rispetto al
% time step precendente, 0 altrienti
coder.extrinsic('evalin', 'wgs84Ellipsoid', 'geodetic2ned');
nogps_lat = 0;
nogps_lon = 0;
[nogps_lat, nogps_lon, ~] = geodetic2ned(...
											0, 0, 0,...
											ned_origin(1), ned_origin(2), ned_origin(3),...
											wgs84Ellipsoid);


if (gps_now(1)==nogps_lat && gps_now(2)==nogps_lon)
	%gps non funzionante
	y = 0;
elseif norm(u) == 0
    y = 0;
else
    y = 1;
end



end

== matlab function TeamA_PAsqualo/Navigazione/Selettore Misure/Selettore misure/pulse2/MATLAB Function ==
  data: u input; y output
function y  = tolo_pulse(u)
% questa funzione fornisce 1 se il valore in ingresso e` cambiato rispetto al
% time step precendente, 0 altrienti

if norm(u) == 0
    y = 0;
else
    y = 1;
end

end

== matlab function TeamA_PAsqualo/Navigazione/Selettore Misure/Selettore misure/pulse4/MATLAB Function ==
  data: u input; y output
function y  = tolo_pulse(u)
% questa funzione fornisce 1 se il valore in ingresso e` cambiato rispetto al
% time step precendente, 0 altrienti

if norm(u) == 0
    y = 0;
else
    y = 1;
end

end

== matlab function TeamA_PAsqualo/Navigazione/dvl2body ==
  data: ni_dvl input; ni output; omega input; p_dvl parameter
function ni = fondcine(ni_dvl, omega, p_dvl)

% dist_dvl_body e` il vettore che va dall'origine del sistema di riferimento 
% body al sensore dvl
 
ni = ni_dvl + cross(omega, -p_dvl);


end

== matlab function TeamA_PAsqualo/Navigazione/geo2ned1 ==
  data: geo input; ned output size=[3 1]; ned_origin parameter
function ned = geo2ned(geo, ned_origin)
coder.extrinsic('evalin', 'wgs84Ellipsoid', 'geodetic2ned');

[x, y, z] = geodetic2ned(geo(1), geo(2), geo(3),ned_origin(1), ned_origin(2), ned_origin(3), wgs84Ellipsoid);

ned = zeros(3,1);
ned = [x;y;z];
end

== matlab function TeamA_PAsqualo/Navigazione/geo2ned2 ==
  data: ned input; LLD output size=[3 1]; ned_origin parameter
function LLD = ned2lld(ned, ned_origin)
coder.extrinsic('evalin', 'wgs84Ellipsoid', 'ned2geodetic');

[Lat, Lon, z] = ned2geodetic(ned(1), ned(2), 0,ned_origin(1), ned_origin(2), ned_origin(3), wgs84Ellipsoid);

LLD = zeros(3,1);
LLD = [Lat; Lon; ned(3)];
end

== matlab function TeamA_PAsqualo/controller/compute_if_enable ==
  settings: updateMethod=DISCRETE  sampleTime=0.1
  data: current_state input size=[8 1]; enable output size=[6 1]
function enable = fcn(current_state)
enable = zeros(6,1);
for i = 1:1:length(current_state)
    if (current_state(i) == 1 && i <= 5)
        enable(i) = 1;
    end
    if i > 5
        if (current_state(i) == 1 && i == 7)
            enable = zeros(6,1);
            enable(2) = 1;
        end
        if (current_state(i) == 1 && i == 8)
            enable = zeros(6,1);
            enable(2) = 0;
            enable(6) = 1;
        end
    end
end
end
